simulink model "simulation"  (R2019b)
settings: Solver=ode45  StartTime=0.0  StopTime=10  FixedStep=0.001  RelTol=1e-9  AbsTol=1e-9
undefined symbols (not defined in the file or in its folder): K_int, modelData, MPC, pv0, ref
libraries: model_library x13, vrlib x7, sharedtransform x5, simulink x2
settings Model: PauseTimes=55  Creator=Matt  LastModifiedBy=Watson
settings SolverCC: MaxOrder=1  ZeroCrossAlgorithm=Adaptive
settings DataIOCC: SaveOutput=off  SignalLogging=off  DSMLogging=off  SaveTime=off  ReturnWorkspaceOutputs=off  StateSaveName=state
settings OptimizationCC: DefaultParameterBehavior=Inlined  UseDivisionForNetSlopeComputation=on  UseFloatMulNetSlope=on  InlineInvariantSignals=on  PassReuseOutputArgsAs=Individual arguments  ZeroExternalMemoryAtStartup=off  ZeroInternalMemoryAtStartup=off  NoFixptDivByZeroProtection=on  EfficientFloat2IntCast=on  LifeSpan=1  OptimizeBlockOrder=speed  DifferentSizesBufferReuse=on  EfficientTunableParamExpr=on
settings DebuggingCC: ReadBeforeWriteMsg=DisableAll  WriteAfterWriteMsg=DisableAll  WriteAfterReadMsg=DisableAll  MultiTaskDSMMsg=none  ParameterTunabilityLossMsg=error  RootOutportRequireBusObject=error  StrictBusMsg=ErrorOnBusTreatedAsVector  SFExecutionAtInitializationDiag=none  ArithmeticOperatorsInVariantConditions=warning
settings HardwareCC: ProdBitPerPointer=32  ProdBitPerSizeT=32  ProdBitPerPtrDiffT=32  ProdLargestAtomicInteger=Long  ProdWordSize=32  ProdLongLongMode=on  ProdHWDeviceType=ARM Compatible->ARM 9
settings ModelReferenceCC: UpdateModelReferenceTargets=IfOutOfDate
settings SFSimCC: SFSimEcho=off  SimUseLocalCustomCode=off  MATLABDynamicMemAlloc=off  CustomCodeUndefinedFunction=UseInterfaceOnly
settings RTWCC: SystemTargetFile=ert.tlc  TemplateMakefile=ert_default_tmf  GenerateReport=on  RTWUseLocalCustomCode=off  Toolchain=Microsoft Visual C++ 2015 v14.0 | nmake (64-bit Windows)  BuildConfiguration=Faster Runs  IncludeHyperlinkInReport=on  LaunchReport=on  GenerateTraceInfo=on  GenerateTraceReport=on  GenerateTraceReportSl=on  GenerateTraceReportSf=on  GenerateTraceReportEml=on  GenerateCodeMetricsReport=on
settings CodeAppCC: ForceParamTrailComments=on  IgnoreCustomStorageClasses=off  MaxIdLength=95  OperatorAnnotations=on  SimulinkDataObjDesc=on  SFDataObjDesc=on  CustomSymbolStrGlobalVar=rt$N$M  CustomSymbolStrType=$N$M  CustomSymbolStrFcn=$N$M$F  CustomSymbolStrMacro=$N$M  InsertBlockDesc=on
settings ERTTargetCC: GenerateSampleERTMain=on  IncludeMdlTerminateFcn=off  CombineSignalStateStructs=on  SupportComplex=off  SupportContinuousTime=on  SupportNonInlinedSFcns=on  InlinedParameterPlacement=NonHierarchical  ERTCustomFileTemplate=example_file_process.tlc  ERTFilePackagingFormat=CompactWithDataFile

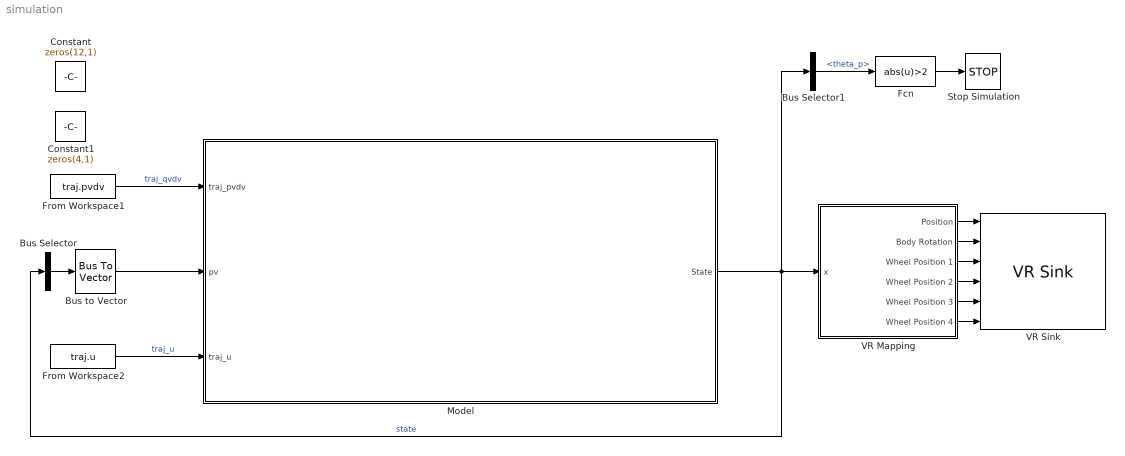
== system simulation ==
  Bus Selector : BusSelector  OutputSignals=x,y,phi,theta_p,vx,vy,dphi,dtheta_p  OutputAsBus=on
  Bus Selector1 : BusSelector  OutputSignals=theta_p
  Bus to Vector : BusToVector
  Constant : Constant  Value=zeros(12,1)
  Constant1 : Constant  Value=zeros(4,1)
  Fcn : Fcn  Expr=abs(u)>2
  From Workspace1 : FromWorkspace  VariableName=traj.pvdv  SampleTime=0  OutputAfterFinalValue=Holding final value
  From Workspace2 : FromWorkspace  VariableName=traj.u  SampleTime=0  OutputAfterFinalValue=Holding final value
  Model : Subsystem
  Stop Simulation : Stop
  VR Mapping : Subsystem
  VR Sink : vrlib/VR Sink  InstantiateOnLoad=on  SampleTime=0.01  ViewEnable=on  RemoteChange=off  RemoteView=off  FieldsWritten=Body_Position.translation.3.1.1.double#Body_Orientation.rotation.4.1.1.double#Wheel4.rotation.4.1.1.double#Wheel3.rotation.4.1.1.double#Wheel2.rotation.4.1.1.double#Wheel1.rotation.4.1.1.double  WorldFileName=3dworld.wrl  AutoView=off  VideoDimensions=[]  AllowVariableSize=off  FigureProperties="{'Position', 'Name', 'Viewpoint', 'CameraBound', 'CameraDirection', 'CameraPosition', 'CameraUpVector', 'ZoomFactor', 'Antialiasing', 'Headlight', 'Lighting', 'NavPanel', 'Sound', 'StatusBar', 'Stereo3D', 'Stereo3DCameraOffset', 'Stereo3DHIT', 'ToolBar', 'Textures', 'Transparency', 'Triad', 'Wireframe', 'NavZones', 'NavMode', 'NavSpeed', 'CaptureFileFormat', 'CaptureFileName', 'Record2DCompressMethod', 'Record2DCompressQuality', 'Record2D', 'Record2DFileName', 'Record2DFPS'; [1.0000000000000000e+00   7.6000000000000000e+01   1.9200000000000000e+03   9.1300000000000000e+02], '', '_untitled_2', 'on', [0.0000000000000000e+00   0.0000000000000000e+00  -1.0000000000000000e+00], [0.0000000000000000e+00   0.0000000000000000e+00   0.0000000000000000e+00], [0.0000000000000000e+00   1.0000000000000000e+00   0.0000000000000000e+00], [1.0000000000000000e+00], 'on', 'on', 'on', 'halfbar', 'on', 'on', 'off', [1.0000000149011612e-01], [0.0000000000000000e+00], 'on', 'on', 'on', 'none', 'off', 'off', 'fly', 'normal', 'tif', '%f_anim_%n.tif', 'auto', [7.5000000000000000e+01], 'off', '%f_anim_%n.avi', 'auto'}"
      settings: SourceProductBaseCode=VR
  wires:
  Model/1(State) -> Bus Selector1/1, VR Mapping/1(x), Bus Selector/1  "state"
  Bus Selector/1 -> Bus to Vector/1
  VR Mapping/1(Position) -> VR Sink/1
  VR Mapping/2(Body Rotation) -> VR Sink/2
  VR Mapping/3(Wheel Position 1) -> VR Sink/3
  VR Mapping/4(Wheel Position 2) -> VR Sink/4
  VR Mapping/5(Wheel Position 3) -> VR Sink/5
  VR Mapping/6(Wheel Position 4) -> VR Sink/6
  Bus to Vector/1 -> Model/2(pv)
  From Workspace1/1 -> Model/1(traj_pvdv)  "traj_qvdv"
  From Workspace2/1 -> Model/3(traj_u)  "traj_u"
  Bus Selector1/1 -> Fcn/1  "<theta_p>"
  Fcn/1 -> Stop Simulation/1

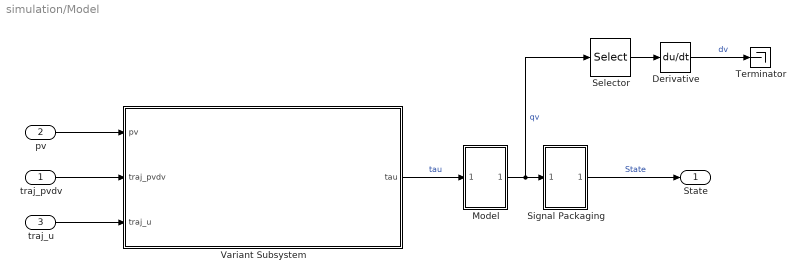
== system simulation/Model ==
  traj_pvdv : Inport
  pv : Inport  Port=2
  traj_u : Inport  Port=3
  Derivative : Derivative
  Model : Subsystem
  Selector : Selector  InputPortWidth=8  IndexOptions=Index vector (dialog)  Indices=[5:8]  OutputSizes=1
  Signal Packaging : Subsystem
  Terminator : Terminator
  Variant Subsystem : Subsystem  VariantControlMode=Label  Variant=on  LabelModeActiveChoice=LQR
  State : Outport  VectorParamsAs1DForOutWhenUnconnected=off
  wires:
  Model/1("[q;v]") -> Selector/1, Signal Packaging/1(In1)  "qv"
  Signal Packaging/1(Out1) -> State/1  "State"
  traj_pvdv/1 -> Variant Subsystem/2(traj_pvdv)
  traj_u/1 -> Variant Subsystem/3(traj_u)
  Selector/1 -> Derivative/1
  Derivative/1 -> Terminator/1  "dv"
  pv/1 -> Variant Subsystem/1(pv)
  Variant Subsystem/1(tau) -> Model/1(tau)  "tau"

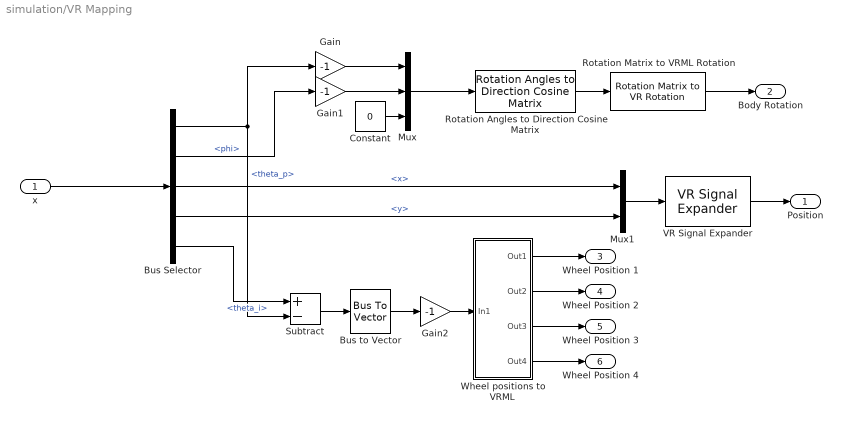
== system simulation/VR Mapping ==
  x : Inport
  Bus Selector : BusSelector  OutputSignals=theta_p,phi,x,y,theta_i
  Bus to Vector : BusToVector
  Constant : Constant  Value=0
  Gain : Gain  Gain=-1
  Gain1 : Gain  Gain=-1
  Gain2 : Gain  Gain=-1
  Mux : Mux  Inputs=3
  Mux1 : Mux  Inputs=2
  Rotation Angles to Direction Cosine Matrix : sharedtransform/Rotation Angles to Direction Cosine Matrix  rotationOrder=XZY  aMode=aMode
      settings: SourceProductBaseCode=AE
  Rotation Matrix to VRML Rotation : vrlib/Utilities/Rotation Matrix to VR Rotation  maxzero=1e-12
      settings: SourceProductName=Simulink 3D Animation  SourceProductBaseCode=VR
  Subtract : Sum  Inputs=+-
  VR Signal Expander : vrlib/VR Signal Expander  outwidth=3  outidx=[1 2]
      settings: SourceProductName=Simulink 3D Animation  SourceProductBaseCode=VR
  Wheel positions to VRML : Subsystem
  Position : Outport  VectorParamsAs1DForOutWhenUnconnected=off
  Body Rotation : Outport  Port=2  VectorParamsAs1DForOutWhenUnconnected=off
  Wheel Position 1 : Outport  Port=3  VectorParamsAs1DForOutWhenUnconnected=off
  Wheel Position 2 : Outport  Port=4  VectorParamsAs1DForOutWhenUnconnected=off
  Wheel Position 3 : Outport  Port=5  VectorParamsAs1DForOutWhenUnconnected=off
  Wheel Position 4 : Outport  Port=6  VectorParamsAs1DForOutWhenUnconnected=off
  wires:
  Mux/1 -> Rotation Angles to Direction Cosine Matrix/1
  Rotation Angles to Direction Cosine Matrix/1 -> Rotation Matrix to VRML Rotation/1
  Rotation Matrix to VRML Rotation/1 -> Body Rotation/1
  Constant/1 -> Mux/3
  VR Signal Expander/1 -> Position/1
  Mux1/1 -> VR Signal Expander/1
  Bus Selector/1 -> Subtract/2, Gain/1  "<theta_p>"
  Bus Selector/2 -> Gain1/1  "<phi>"
  Bus Selector/3 -> Mux1/1  "<x>"
  Bus Selector/4 -> Mux1/2  "<y>"
  Bus to Vector/1 -> Gain2/1
  Subtract/1 -> Bus to Vector/1
  Bus Selector/5 -> Subtract/1  "<theta_i>"
  Gain/1 -> Mux/1
  Gain1/1 -> Mux/2
  Gain2/1 -> Wheel positions to VRML/1(In1)
  x/1 -> Bus Selector/1
  Wheel positions to VRML/1(Out1) -> Wheel Position 1/1
  Wheel positions to VRML/2(Out2) -> Wheel Position 2/1
  Wheel positions to VRML/3(Out3) -> Wheel Position 3/1
  Wheel positions to VRML/4(Out4) -> Wheel Position 4/1

== system simulation/Model/Model ==
  tau : Inport
  Integrator2 : Integrator  InitialCondition=pv0
  dynamics_dqdv : model_library/dynamics_dqdv  SystemSampleTime=-1  Latency=0  AutoFrameSizeCalculation=off
  "[q;v]" : Outport  VectorParamsAs1DForOutWhenUnconnected=off
  wires:
  Integrator2/1 -> dynamics_dqdv/1, "[q;v]"/1
  dynamics_dqdv/1 -> Integrator2/1  "dqdv"
  tau/1 -> dynamics_dqdv/2

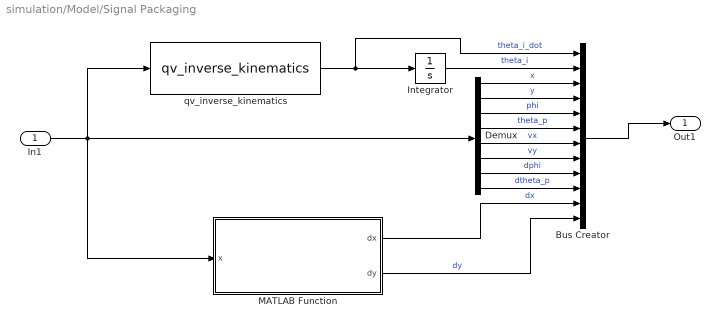
== system simulation/Model/Signal Packaging ==
  In1 : Inport
  Bus Creator : BusCreator  Inputs=12
  Demux : Demux  Outputs=8
  Integrator : Integrator  InitialCondition=[0 0 0 0]
  MATLAB Function : MATLAB Function  TreatAsAtomicUnit=on
  qv_inverse_kinematics : model_library/qv_inverse_kinematics  SystemSampleTime=-1  Latency=0  AutoFrameSizeCalculation=off
  Out1 : Outport  VectorParamsAs1DForOutWhenUnconnected=off
  wires:
  Demux/1 -> Bus Creator/3  "x"
  Demux/6 -> Bus Creator/8  "vy"
  Demux/3 -> Bus Creator/5  "phi"
  Demux/7 -> Bus Creator/9  "dphi"
  qv_inverse_kinematics/1 -> Integrator/1, Bus Creator/1  "theta_i_dot"
  Demux/8 -> Bus Creator/10  "dtheta_p"
  In1/1 -> MATLAB Function/1(x), Demux/1, qv_inverse_kinematics/1
  Demux/2 -> Bus Creator/4  "y"
  Demux/4 -> Bus Creator/6  "theta_p"
  Demux/5 -> Bus Creator/7  "vx"
  Integrator/1 -> Bus Creator/2  "theta_i"
  Bus Creator/1 -> Out1/1
  MATLAB Function/1(dx) -> Bus Creator/11  "dx"
  MATLAB Function/2(dy) -> Bus Creator/12  "dy"

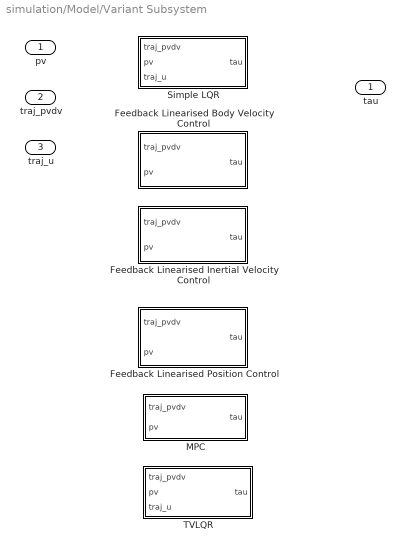
== system simulation/Model/Variant Subsystem ==
  pv : Inport
  traj_pvdv : Inport  Port=2
  traj_u : Inport  Port=3
  Feedback Linearised Body Velocity Control : Subsystem  VariantControl=FeedbackLinearisedBodyVelocity
  Feedback Linearised Inertial Velocity Control : Subsystem  VariantControl=FeedbackLinearisedInertialVelocity
  Feedback Linearised Position Control : Subsystem  VariantControl=FeedbackLinearisedPosition
  MPC : Subsystem  VariantControl=Variant
  Simple LQR : Subsystem  VariantControl=LQR
  TVLQR : Subsystem  VariantControl=TVLQR
  tau : Outport  VectorParamsAs1DForOutWhenUnconnected=off

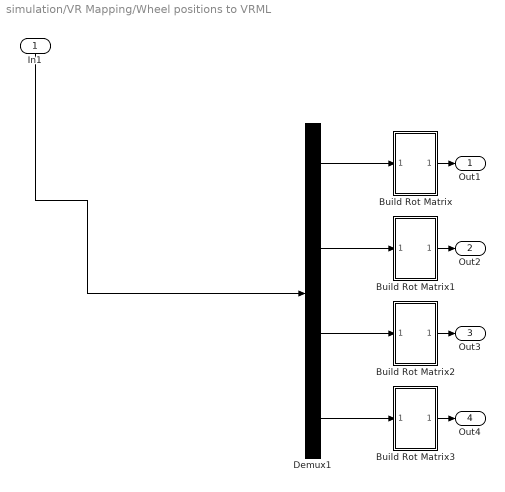
== system simulation/VR Mapping/Wheel positions to VRML ==
  In1 : Inport
  Build Rot Matrix : Subsystem
  Build Rot Matrix1 : Subsystem
  Build Rot Matrix2 : Subsystem
  Build Rot Matrix3 : Subsystem
  Demux1 : Demux
  Out1 : Outport  VectorParamsAs1DForOutWhenUnconnected=off
  Out2 : Outport  Port=2  VectorParamsAs1DForOutWhenUnconnected=off
  Out3 : Outport  Port=3  VectorParamsAs1DForOutWhenUnconnected=off
  Out4 : Outport  Port=4  VectorParamsAs1DForOutWhenUnconnected=off
  wires:
  Demux1/3 -> Build Rot Matrix2/1(In1)
  Build Rot Matrix1/1(Out1) -> Out2/1
  Build Rot Matrix3/1(Out1) -> Out4/1
  Build Rot Matrix2/1(Out1) -> Out3/1
  In1/1 -> Demux1/1
  Demux1/2 -> Build Rot Matrix1/1(In1)
  Demux1/4 -> Build Rot Matrix3/1(In1)
  Demux1/1 -> Build Rot Matrix/1(In1)
  Build Rot Matrix/1(Out1) -> Out1/1

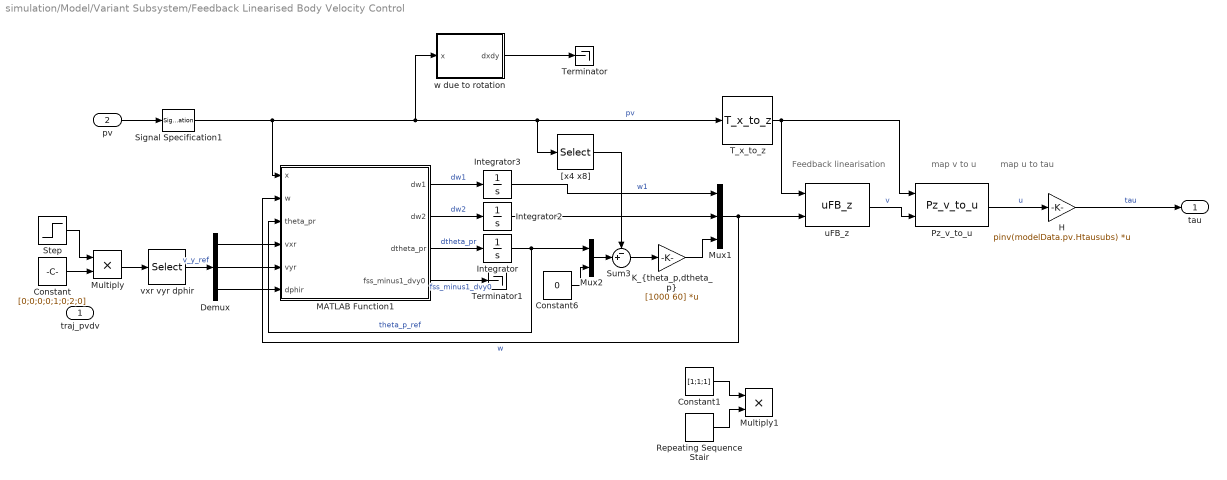
== system simulation/Model/Variant Subsystem/Feedback Linearised Body Velocity Control ==
  note: Feedback linearisation
  note: map v to u
  note: map u to tau
  traj_pvdv : Inport
  pv : Inport  Port=2
  Constant : Constant  Value=[0;0;0;0;1;0;2;0]
  Constant1 : Constant  Value=[1;1;1]
  Constant6 : Constant  Value=0
  Demux : Demux  Outputs=3
  H : Gain  Gain=pinv(modelData.pv.Htausubs)  Multiplication=Matrix(K*u)
  Integrator : Integrator  InitialCondition=pv0(4)
  Integrator2 : Integrator
  Integrator3 : Integrator
  "K_{theta_p,dtheta_p}" : Gain  Gain=[1000 60]  Multiplication=Matrix(K*u)
  MATLAB Function1 : MATLAB Function  TreatAsAtomicUnit=on
  Multiply : Product
  Multiply1 : Product
  Mux1 : Mux  Inputs=3
  Mux2 : Mux  Inputs=2
  Pz_v_to_u : model_library/Pz_v_to_u  SystemSampleTime=-1  Latency=0  AutoFrameSizeCalculation=off
  Repeating Sequence Stair : simulink/Sources/Repeating Sequence Stair  OutValues=[1 -1 -1 1]  tsamp=1  OutMin=[]  OutMax=[]  OutDataTypeStr=double  OutputDataTypeScalingMode=double  OutDataType=fixdt(0,8)  ConRadixGroup=Best Precision: Vector-wise  OutScaling=2^-12
  Signal Specification1 : SignalSpecification  Dimensions=[8 1]
  Step : Step  SampleTime=0
  Sum3 : Sum  Inputs=-+|
  T_x_to_z : model_library/T_x_to_z  SystemSampleTime=-1  Latency=0  AutoFrameSizeCalculation=off
  Terminator : Terminator
  Terminator1 : Terminator
  "[x4 x8]" : Selector  InputPortWidth=8  IndexOptions=Index vector (dialog)  Indices=[4 8]  OutputSizes=1
  uFB_z : model_library/uFB_z  SystemSampleTime=-1  Latency=0  AutoFrameSizeCalculation=off
  vxr vyr dphir : Selector  InputPortWidth=8  IndexOptions=Index vector (dialog)  Indices=5:7  OutputSizes=1
  w due to rotation : MATLAB Function  TreatAsAtomicUnit=on
  tau : Outport  VectorParamsAs1DForOutWhenUnconnected=off
  wires:
  T_x_to_z/1 -> uFB_z/1, Pz_v_to_u/1
  Sum3/1 -> "K_{theta_p,dtheta_p}"/1
  uFB_z/1 -> Pz_v_to_u/2  "v"
  "[x4 x8]"/1 -> Sum3/1
  pv/1 -> Signal Specification1/1
  Signal Specification1/1 -> MATLAB Function1/1(x), w due to rotation/1(x), T_x_to_z/1, "[x4 x8]"/1  "pv"
  H/1 -> tau/1  "tau"
  Mux2/1 -> Sum3/2
  Demux/2 -> MATLAB Function1/5(vyr)
  Demux/1 -> MATLAB Function1/4(vxr)
  Demux/3 -> MATLAB Function1/6(dphir)
  vxr vyr dphir/1 -> Demux/1  "v_y_ref"
  MATLAB Function1/3(dtheta_pr) -> Integrator/1  "dtheta_pr"
  MATLAB Function1/1(dw1) -> Integrator3/1  "dw1"
  MATLAB Function1/2(dw2) -> Integrator2/1  "dw2"
  "K_{theta_p,dtheta_p}"/1 -> Mux1/3
  Pz_v_to_u/1 -> H/1  "u"
  Integrator2/1 -> Mux1/2
  Mux1/1 -> uFB_z/2, MATLAB Function1/2(w)  "w"
  Constant6/1 -> Mux2/2
  Integrator3/1 -> Mux1/1  "w1"
  Integrator/1 -> MATLAB Function1/3(theta_pr), Mux2/1  "theta_p_ref"
  w due to rotation/1(dxdy) -> Terminator/1
  MATLAB Function1/4(fss_minus1_dvy0) -> Terminator1/1  "fss_minus1_dvy0"
  Constant/1 -> Multiply/2
  Multiply/1 -> vxr vyr dphir/1
  Step/1 -> Multiply/1
  Repeating Sequence Stair/1 -> Multiply1/2
  Constant1/1 -> Multiply1/1

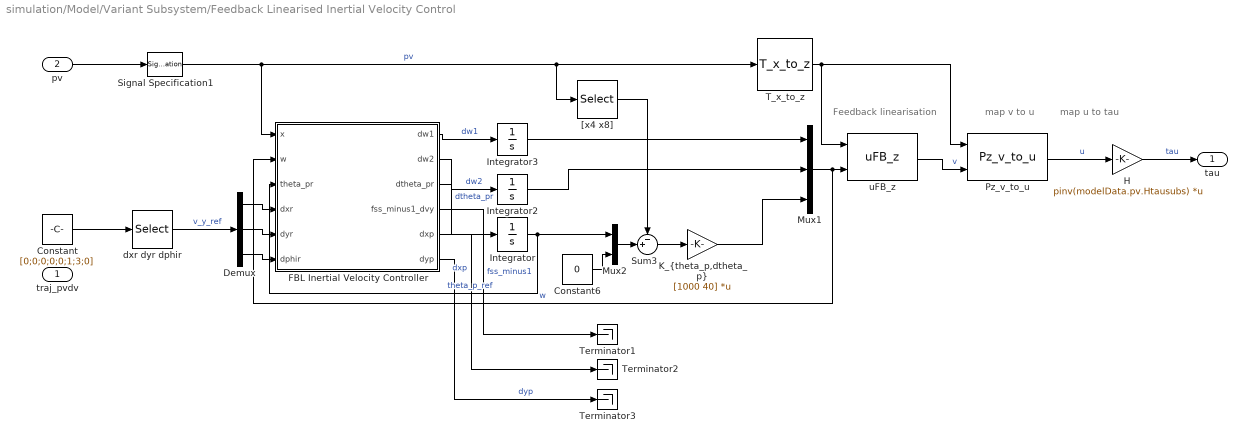
== system simulation/Model/Variant Subsystem/Feedback Linearised Inertial Velocity Control ==
  note: Feedback linearisation
  note: map v to u
  note: map u to tau
  traj_pvdv : Inport
  pv : Inport  Port=2
  Constant : Constant  Value=[0;0;0;0;0;1;3;0]
  Constant6 : Constant  Value=0
  Demux : Demux  Outputs=3
  FBL Inertial Velocity Controller : MATLAB Function  TreatAsAtomicUnit=on
  H : Gain  Gain=pinv(modelData.pv.Htausubs)  Multiplication=Matrix(K*u)
  Integrator : Integrator
  Integrator2 : Integrator
  Integrator3 : Integrator
  "K_{theta_p,dtheta_p}" : Gain  Gain=[1000 40]  Multiplication=Matrix(K*u)
  Mux1 : Mux  Inputs=3
  Mux2 : Mux  Inputs=2
  Pz_v_to_u : model_library/Pz_v_to_u  SystemSampleTime=-1  Latency=0  AutoFrameSizeCalculation=off
  Signal Specification1 : SignalSpecification  Dimensions=[8 1]
  Sum3 : Sum  Inputs=-+|
  T_x_to_z : model_library/T_x_to_z  SystemSampleTime=-1  Latency=0  AutoFrameSizeCalculation=off
  Terminator1 : Terminator
  Terminator2 : Terminator
  Terminator3 : Terminator
  "[x4 x8]" : Selector  InputPortWidth=8  IndexOptions=Index vector (dialog)  Indices=[4 8]  OutputSizes=1
  dxr dyr dphir : Selector  InputPortWidth=8  IndexOptions=Index vector (dialog)  Indices=5:7  OutputSizes=1
  uFB_z : model_library/uFB_z  SystemSampleTime=-1  Latency=0  AutoFrameSizeCalculation=off
  tau : Outport  VectorParamsAs1DForOutWhenUnconnected=off
  wires:
  T_x_to_z/1 -> uFB_z/1, Pz_v_to_u/1
  Sum3/1 -> "K_{theta_p,dtheta_p}"/1
  "[x4 x8]"/1 -> Sum3/1
  pv/1 -> Signal Specification1/1
  Signal Specification1/1 -> T_x_to_z/1, "[x4 x8]"/1, FBL Inertial Velocity Controller/1(x)  "pv"
  H/1 -> tau/1  "tau"
  Mux2/1 -> Sum3/2
  Constant/1 -> dxr dyr dphir/1
  Demux/2 -> FBL Inertial Velocity Controller/5(dyr)
  Demux/1 -> FBL Inertial Velocity Controller/4(dxr)
  Demux/3 -> FBL Inertial Velocity Controller/6(dphir)
  dxr dyr dphir/1 -> Demux/1  "v_y_ref"
  FBL Inertial Velocity Controller/2(dw2) -> Integrator2/1  "dw2"
  FBL Inertial Velocity Controller/1(dw1) -> Integrator3/1  "dw1"
  Mux1/1 -> FBL Inertial Velocity Controller/2(w), uFB_z/2  "w"
  uFB_z/1 -> Pz_v_to_u/2  "v"
  Pz_v_to_u/1 -> H/1  "u"
  Integrator2/1 -> Mux1/2
  Integrator3/1 -> Mux1/1
  FBL Inertial Velocity Controller/3(dtheta_pr) -> Integrator/1  "dtheta_pr"
  "K_{theta_p,dtheta_p}"/1 -> Mux1/3
  Integrator/1 -> FBL Inertial Velocity Controller/3(theta_pr), Mux2/1  "theta_p_ref"
  Constant6/1 -> Mux2/2
  FBL Inertial Velocity Controller/4(fss_minus1_dvy) -> Terminator1/1  "fss_minus1"
  FBL Inertial Velocity Controller/5(dxp) -> Terminator2/1  "dxp"
  FBL Inertial Velocity Controller/6(dyp) -> Terminator3/1  "dyp"

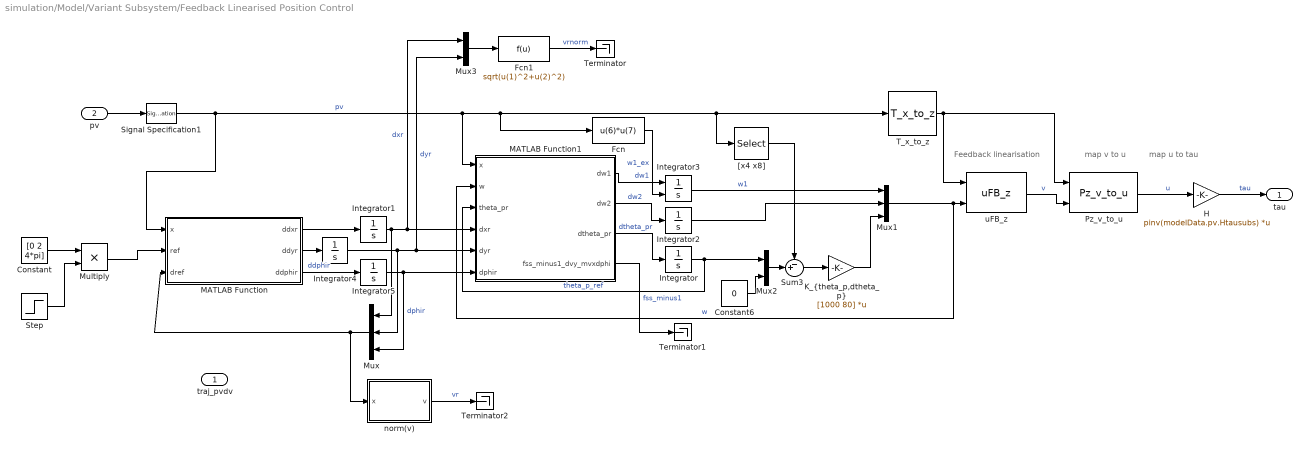
== system simulation/Model/Variant Subsystem/Feedback Linearised Position Control ==
  note: Feedback linearisation
  note: map v to u
  note: map u to tau
  traj_pvdv : Inport
  pv : Inport  Port=2
  Constant : Constant  Value=[0 2 4*pi]
  Constant6 : Constant  Value=0
  Fcn : Fcn  Expr=u(6)*u(7)
  Fcn1 : Fcn  Expr=sqrt(u(1)^2+u(2)^2)
  H : Gain  Gain=pinv(modelData.pv.Htausubs)  Multiplication=Matrix(K*u)
  Integrator : Integrator  InitialCondition=pv0(4)
  Integrator{1..2,4..5} (4 alike) : Integrator
  Integrator3 : Integrator  InitialConditionSource=external
  "K_{theta_p,dtheta_p}" : Gain  Gain=[1000 80]  Multiplication=Matrix(K*u)
  MATLAB Function : MATLAB Function  TreatAsAtomicUnit=on
  MATLAB Function1 : MATLAB Function  TreatAsAtomicUnit=on
  Multiply : Product
  Mux : Mux  Inputs=3
  Mux1 : Mux  Inputs=3
  Mux2 : Mux  Inputs=2
  Mux3 : Mux  Inputs=2
  Pz_v_to_u : model_library/Pz_v_to_u  SystemSampleTime=-1  Latency=0  AutoFrameSizeCalculation=off
  Signal Specification1 : SignalSpecification  Dimensions=[8 1]
  Step : Step  Time=2  SampleTime=0
  Sum3 : Sum  Inputs=-+|
  T_x_to_z : model_library/T_x_to_z  SystemSampleTime=-1  Latency=0  AutoFrameSizeCalculation=off
  Terminator : Terminator
  Terminator1 : Terminator
  Terminator2 : Terminator
  "[x4 x8]" : Selector  InputPortWidth=8  IndexOptions=Index vector (dialog)  Indices=[4 8]  OutputSizes=1
  norm(v) : MATLAB Function  TreatAsAtomicUnit=on
  uFB_z : model_library/uFB_z  SystemSampleTime=-1  Latency=0  AutoFrameSizeCalculation=off
  tau : Outport  VectorParamsAs1DForOutWhenUnconnected=off
  wires:
  MATLAB Function/1(ddxr) -> Integrator1/1
  MATLAB Function/3(ddphir) -> Integrator5/1  "ddphir"
  Integrator2/1 -> Mux1/2
  "[x4 x8]"/1 -> Sum3/1
  uFB_z/1 -> Pz_v_to_u/2  "v"
  Sum3/1 -> "K_{theta_p,dtheta_p}"/1
  T_x_to_z/1 -> uFB_z/1, Pz_v_to_u/1
  Signal Specification1/1 -> MATLAB Function/1(x), T_x_to_z/1, "[x4 x8]"/1, Fcn/1, MATLAB Function1/1(x)  "pv"
  MATLAB Function1/2(dw2) -> Integrator2/1  "dw2"
  "K_{theta_p,dtheta_p}"/1 -> Mux1/3
  H/1 -> tau/1  "tau"
  Fcn/1 -> Integrator3/2  "w1_ex"
  Integrator3/1 -> Mux1/1  "w1"
  pv/1 -> Signal Specification1/1
  Pz_v_to_u/1 -> H/1  "u"
  Integrator/1 -> MATLAB Function1/3(theta_pr), Mux2/1  "theta_p_ref"
  Mux2/1 -> Sum3/2
  MATLAB Function1/1(dw1) -> Integrator3/1  "dw1"
  Constant6/1 -> Mux2/2
  Mux1/1 -> MATLAB Function1/2(w), uFB_z/2  "w"
  MATLAB Function1/3(dtheta_pr) -> Integrator/1  "dtheta_pr"
  MATLAB Function/2(ddyr) -> Integrator4/1
  Integrator1/1 -> Mux/1, Mux3/1, MATLAB Function1/4(dxr)  "dxr"
  Integrator4/1 -> Mux/2, Mux3/2, MATLAB Function1/5(dyr)  "dyr"
  Integrator5/1 -> Mux/3, MATLAB Function1/6(dphir)  "dphir"
  Fcn1/1 -> Terminator/1  "vrnorm"
  Mux3/1 -> Fcn1/1
  MATLAB Function1/4(fss_minus1_dvy_mvxdphi) -> Terminator1/1  "fss_minus1"
  Mux/1 -> norm(v)/1(x), MATLAB Function/3(dref)
  norm(v)/1(v) -> Terminator2/1  "vr"
  Constant/1 -> Multiply/1
  Step/1 -> Multiply/2
  Multiply/1 -> MATLAB Function/2(ref)

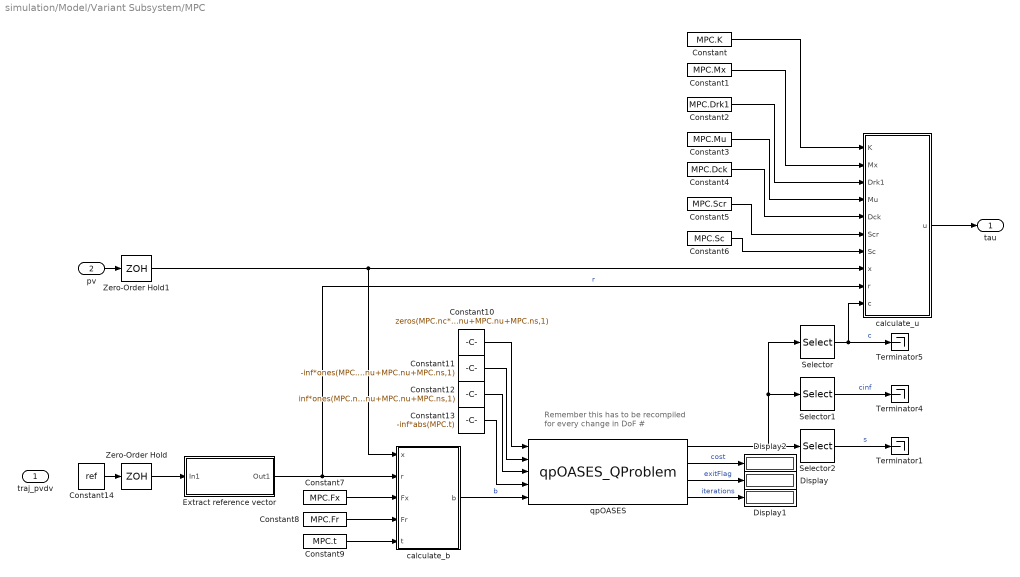
== system simulation/Model/Variant Subsystem/MPC ==
  note: Remember this has to be recompiled
      | for every change in DoF #
  traj_pvdv : Inport
  pv : Inport  Port=2
  Constant : Constant  Value=MPC.K
  Constant1 : Constant  Value=MPC.Mx
  Constant10 : Constant  Value=zeros(MPC.nc*MPC.nu+MPC.nu+MPC.ns,1)
  Constant11 : Constant  Value=-inf*ones(MPC.nc*MPC.nu+MPC.nu+MPC.ns,1)
  Constant12 : Constant  Value=inf*ones(MPC.nc*MPC.nu+MPC.nu+MPC.ns,1)
  Constant13 : Constant  Value=-inf*abs(MPC.t)
  Constant14 : Constant  Value=ref
  Constant2 : Constant  Value=MPC.Drk1
  Constant3 : Constant  Value=MPC.Mu
  Constant4 : Constant  Value=MPC.Dck
  Constant5 : Constant  Value=MPC.Scr
  Constant6 : Constant  Value=MPC.Sc
  Constant7 : Constant  Value=MPC.Fx
  Constant8 : Constant  Value=MPC.Fr
  Constant9 : Constant  Value=MPC.t
  Display : Display
  Display1 : Display
  Display2 : Display
  Extract reference vector : Subsystem
  Selector : Selector  InputPortWidth=MPC.nc*MPC.nu + MPC.nu + MPC.ns  IndexOptions=Index vector (dialog)  Indices=[1:MPC.nc*MPC.nu]  OutputSizes=1
  Selector1 : Selector  InputPortWidth=MPC.nc*MPC.nu + MPC.nu + MPC.ns  IndexOptions=Index vector (dialog)  Indices=[1+MPC.nc*MPC.nu:MPC.nc*MPC.nu+MPC.nu]  OutputSizes=1
  Selector2 : Selector  InputPortWidth=MPC.nc*MPC.nu + MPC.nu + MPC.ns  IndexOptions=Index vector (dialog)  Indices=[1+MPC.nc*MPC.nu+MPC.nu:MPC.nc*MPC.nu+MPC.nu+MPC.ns]  OutputSizes=1
  Terminator1 : Terminator
  Terminator4 : Terminator
  Terminator5 : Terminator
  Zero-Order Hold : ZeroOrderHold  SampleTime=MPC.Ts
  Zero-Order Hold1 : ZeroOrderHold  SampleTime=MPC.Ts
  calculate_b : MATLAB Function  TreatAsAtomicUnit=on
  calculate_u : MATLAB Function  TreatAsAtomicUnit=on
  qpOASES : S-Function  FunctionName=qpOASES_QProblem  Parameters=MPC.H,MPC.A  SFunctionDeploymentMode=off  EnableBusSupport=off
  tau : Outport  VectorParamsAs1DForOutWhenUnconnected=off
  wires:
  Constant13/1 -> qpOASES/4
  Constant2/1 -> calculate_u/3(Drk1)
  Constant3/1 -> calculate_u/4(Mu)
  Constant11/1 -> qpOASES/2
  Extract reference vector/1(Out1) -> calculate_u/9(r), calculate_b/2(r)  "r"
  qpOASES/2 -> Display2/1  "cost"
  Constant4/1 -> calculate_u/5(Dck)
  Selector1/1 -> Terminator4/1  "cinf"
  calculate_u/1(u) -> tau/1
  Constant10/1 -> qpOASES/1
  calculate_b/1(b) -> qpOASES/5  "b"
  Constant7/1 -> calculate_b/3(Fx)
  Constant1/1 -> calculate_u/2(Mx)
  Constant8/1 -> calculate_b/4(Fr)
  qpOASES/3 -> Display/1  "exitFlag"
  Constant/1 -> calculate_u/1(K)
  Constant6/1 -> calculate_u/7(Sc)
  qpOASES/4 -> Display1/1  "iterations"
  qpOASES/1 -> Selector2/1, Selector1/1, Selector/1
  Constant5/1 -> calculate_u/6(Scr)
  Selector/1 -> Terminator5/1, calculate_u/10(c)  "c"
  Selector2/1 -> Terminator1/1  "s"
  pv/1 -> Zero-Order Hold1/1
  Constant12/1 -> qpOASES/3
  Constant9/1 -> calculate_b/5(t)
  Constant14/1 -> Zero-Order Hold/1
  Zero-Order Hold/1 -> Extract reference vector/1(In1)
  Zero-Order Hold1/1 -> calculate_b/1(x), calculate_u/8(x)

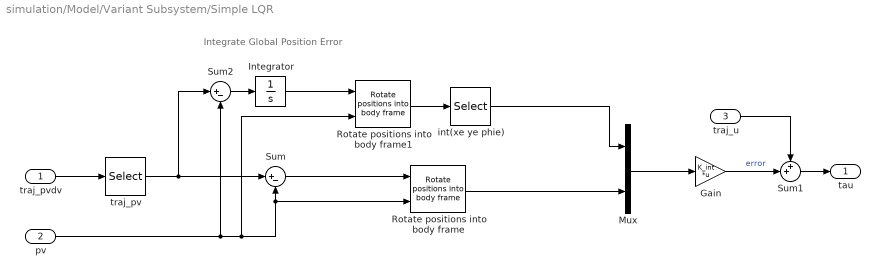
== system simulation/Model/Variant Subsystem/Simple LQR ==
  note: Integrate Global Position Error
  traj_pvdv : Inport
  pv : Inport  Port=2
  traj_u : Inport  Port=3
  Gain : Gain  Gain=K_int  Multiplication=Matrix(K*u)
  Integrator : Integrator  InitialCondition=zeros(8,1)
  Mux : Mux  Inputs=2
  Rotate positions into body frame : model_library/Rotate positions into body frame  SystemSampleTime=-1  Latency=0  AutoFrameSizeCalculation=off
  Rotate positions into body frame1 : model_library/Rotate positions into body frame  SystemSampleTime=-1  Latency=0  AutoFrameSizeCalculation=off
  Sum : Sum  Inputs=|+-
  Sum1 : Sum  Inputs=++|
  Sum2 : Sum  Inputs=|+-
  int(xe ye phie) : Selector  InputPortWidth=8  IndexOptions=Index vector (dialog)  Indices=[1:3]  OutputSizes=1
  traj_pv : Selector  InputPortWidth=12  IndexOptions=Index vector (dialog)  Indices=[1:8]  OutputSizes=1
  tau : Outport  VectorParamsAs1DForOutWhenUnconnected=off
  wires:
  Gain/1 -> Sum1/2  "error"
  traj_u/1 -> Sum1/1
  Sum1/1 -> tau/1
  Sum/1 -> Rotate positions into body frame/1
  Sum2/1 -> Integrator/1
  Rotate positions into body frame1/1 -> int(xe ye phie)/1
  Integrator/1 -> Rotate positions into body frame1/1
  Rotate positions into body frame/1 -> Mux/2
  int(xe ye phie)/1 -> Mux/1
  traj_pvdv/1 -> traj_pv/1
  pv/1 -> Rotate positions into body frame1/2, Rotate positions into body frame/2, Sum/2, Sum2/2
  Mux/1 -> Gain/1
  traj_pv/1 -> Sum2/1, Sum/1

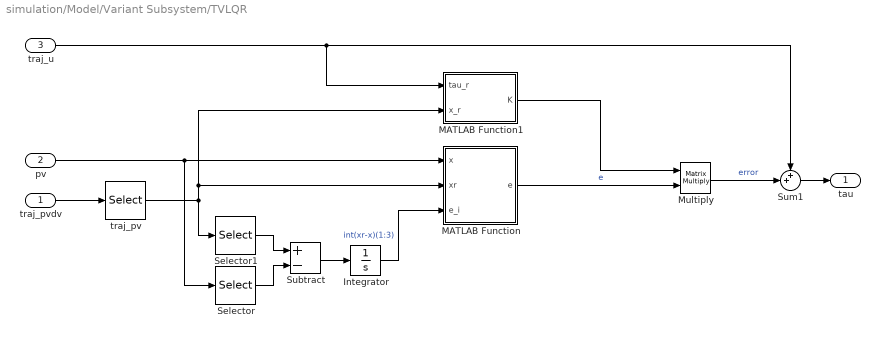
== system simulation/Model/Variant Subsystem/TVLQR ==
  traj_pvdv : Inport
  pv : Inport  Port=2
  traj_u : Inport  Port=3
  Integrator : Integrator  InitialCondition=zeros(3,1)
  MATLAB Function : MATLAB Function  TreatAsAtomicUnit=on
  MATLAB Function1 : MATLAB Function  TreatAsAtomicUnit=on  SystemSampleTime=0.01
  Multiply : Product  Multiplication=Matrix(*)
  Selector : Selector  InputPortWidth=8  IndexOptions=Index vector (dialog)  Indices=[1:3]  OutputSizes=1
  Selector1 : Selector  InputPortWidth=8  IndexOptions=Index vector (dialog)  Indices=[1:3]  OutputSizes=1
  Subtract : Sum  Inputs=+-
  Sum1 : Sum  Inputs=++|
  traj_pv : Selector  InputPortWidth=12  IndexOptions=Index vector (dialog)  Indices=[1:8]  OutputSizes=1
  tau : Outport  VectorParamsAs1DForOutWhenUnconnected=off
  wires:
  Multiply/1 -> Sum1/2  "error"
  Sum1/1 -> tau/1
  traj_pvdv/1 -> traj_pv/1
  pv/1 -> MATLAB Function/1(x), Selector/1
  traj_pv/1 -> Selector1/1, MATLAB Function1/2(x_r), MATLAB Function/2(xr)
  traj_u/1 -> MATLAB Function1/1(tau_r), Sum1/1
  MATLAB Function1/1(K) -> Multiply/1
  MATLAB Function/1(e) -> Multiply/2  "e"
  Selector1/1 -> Subtract/1
  Selector/1 -> Subtract/2
  Subtract/1 -> Integrator/1
  Integrator/1 -> MATLAB Function/3(e_i)  "int(xr-x)(1:3)"

== system simulation/VR Mapping/Wheel positions to VRML/Build Rot Matrix ==
  In1 : Inport
  Constant1 : Constant  Value=pi/2
  Constant2 : Constant  Value=pi/2
  Mux : Mux  Inputs=3
  Rotation Angles to Direction Cosine Matrix : sharedtransform/Rotation Angles to Direction Cosine Matrix  rotationOrder=YZX  aMode=aMode
      settings: SourceProductBaseCode=AE
  Rotation Matrix to VRML Rotation1 : vrlib/Utilities/Rotation Matrix to VR Rotation  maxzero=1e-12
      settings: SourceProductName=Simulink 3D Animation  SourceProductBaseCode=VR
  Out1 : Outport  VectorParamsAs1DForOutWhenUnconnected=off
  wires:
  In1/1 -> Mux/1
  Mux/1 -> Rotation Angles to Direction Cosine Matrix/1
  Constant1/1 -> Mux/2
  Constant2/1 -> Mux/3
  Rotation Angles to Direction Cosine Matrix/1 -> Rotation Matrix to VRML Rotation1/1
  Rotation Matrix to VRML Rotation1/1 -> Out1/1

== system simulation/VR Mapping/Wheel positions to VRML/Build Rot Matrix1 ==
  In1 : Inport
  Constant1 : Constant  Value=pi/2
  Constant2 : Constant  Value=pi/2
  Mux : Mux  Inputs=3
  Rotation Angles to Direction Cosine Matrix : sharedtransform/Rotation Angles to Direction Cosine Matrix  rotationOrder=YZX  aMode=aMode
      settings: SourceProductBaseCode=AE
  Rotation Matrix to VRML Rotation1 : vrlib/Utilities/Rotation Matrix to VR Rotation  maxzero=1e-12
      settings: SourceProductName=Simulink 3D Animation  SourceProductBaseCode=VR
  Out1 : Outport  VectorParamsAs1DForOutWhenUnconnected=off
  wires:
  In1/1 -> Mux/1
  Mux/1 -> Rotation Angles to Direction Cosine Matrix/1
  Constant1/1 -> Mux/2
  Constant2/1 -> Mux/3
  Rotation Angles to Direction Cosine Matrix/1 -> Rotation Matrix to VRML Rotation1/1
  Rotation Matrix to VRML Rotation1/1 -> Out1/1

== system simulation/VR Mapping/Wheel positions to VRML/Build Rot Matrix2 ==
  In1 : Inport
  Constant1 : Constant  Value=pi/2
  Constant2 : Constant  Value=pi/2
  Mux : Mux  Inputs=3
  Rotation Angles to Direction Cosine Matrix : sharedtransform/Rotation Angles to Direction Cosine Matrix  rotationOrder=YZX  aMode=aMode
      settings: SourceProductBaseCode=AE
  Rotation Matrix to VRML Rotation1 : vrlib/Utilities/Rotation Matrix to VR Rotation  maxzero=1e-12
      settings: SourceProductName=Simulink 3D Animation  SourceProductBaseCode=VR
  Out1 : Outport  VectorParamsAs1DForOutWhenUnconnected=off
  wires:
  In1/1 -> Mux/1
  Mux/1 -> Rotation Angles to Direction Cosine Matrix/1
  Constant1/1 -> Mux/2
  Constant2/1 -> Mux/3
  Rotation Angles to Direction Cosine Matrix/1 -> Rotation Matrix to VRML Rotation1/1
  Rotation Matrix to VRML Rotation1/1 -> Out1/1

== system simulation/VR Mapping/Wheel positions to VRML/Build Rot Matrix3 ==
  In1 : Inport
  Constant1 : Constant  Value=pi/2
  Constant2 : Constant  Value=pi/2
  Mux : Mux  Inputs=3
  Rotation Angles to Direction Cosine Matrix : sharedtransform/Rotation Angles to Direction Cosine Matrix  rotationOrder=YZX  aMode=aMode
      settings: SourceProductBaseCode=AE
  Rotation Matrix to VRML Rotation1 : vrlib/Utilities/Rotation Matrix to VR Rotation  maxzero=1e-12
      settings: SourceProductName=Simulink 3D Animation  SourceProductBaseCode=VR
  Out1 : Outport  VectorParamsAs1DForOutWhenUnconnected=off
  wires:
  In1/1 -> Mux/1
  Mux/1 -> Rotation Angles to Direction Cosine Matrix/1
  Constant1/1 -> Mux/2
  Constant2/1 -> Mux/3
  Rotation Angles to Direction Cosine Matrix/1 -> Rotation Matrix to VRML Rotation1/1
  Rotation Matrix to VRML Rotation1/1 -> Out1/1

== system simulation/Model/Variant Subsystem/MPC/Extract reference vector ==
  In1 : Inport
  Increment Stored Integer : simulink/Additional Math & Discrete/Additional Math: Increment - Decrement/Increment Stored Integer
      settings: SourceProductName=Simulink
  Reshape : Reshape  OutputDimensions=1
  Selector : Selector  NumberOfDimensions=2  InputPortWidth=3  IndexOptions=Select all,Starting index (port)  Indices=[1 3],1  OutputSizes=1,MPC.nr
  Unit Delay : UnitDelay  InitialCondition=1  SampleTime=MPC.Ts  HasFrameUpgradeWarning=on
  Out1 : Outport  VectorParamsAs1DForOutWhenUnconnected=off
  wires:
  In1/1 -> Selector/1
  Unit Delay/1 -> Selector/2, Increment Stored Integer/1
  Increment Stored Integer/1 -> Unit Delay/1
  Selector/1 -> Reshape/1
  Reshape/1 -> Out1/1

== matlab function simulation/Model/Signal Packaging/MATLAB Function ==
  data: x input; dx output; dy output
function [dx,dy] = body_to_inertial_velocities(x)

phi = x(3);
R_EB = [cos(phi) -sin(phi);
            sin(phi) cos(phi)];

dxdy = R_EB*[x(5);x(6)];

dx = dxdy(1);
dy = dxdy(2);

== matlab function simulation/Model/Variant Subsystem/Feedback Linearised Position Control/MATLAB Function1 ==
  data: dw1 output; dw2 output; x input; w input; dtheta_pr output; theta_pr input; dxr input; dyr input; dphir input; fss_minus1_dvy_mvxdphi output
function [dw1,dw2,dtheta_pr,fss_minus1_dvy_mvxdphi] = get_dtheta_pr_dw1_dw2(x, w, theta_pr, dxr, dyr, dphir)

dw1 = 0;
dw2 = 0;
dtheta_pr = 0;
dvy_ss = 0;
fss_minus1_dvy_mvxdphi = 0;
theta_p_ss_error = 0;
% w1_0 = x(6)*x(7);


K_slow_dtheta_p = 0;
K_slow_theta_p = 20;
Kv = 6;
Kdphi = 0.1;

Kr = -150;
Kw1 = 50;
Kw2 = 150;

theta_p_max = 0.4;
w1_max = 3;
w2_max = 15;


% Calculate vxr vyr
phi = x(3);
R_EB = [cos(phi) -sin(phi);
            sin(phi) cos(phi)];
        
vxrvyr = R_EB'*[dxr;dyr];
vxr = vxrvyr(1);
vyr = vxrvyr(2);


% Calculate target steady state theta_p value for dvy=0 - remember this doesnt depend on v_y
fun = @(toSolve) f_solve_fdvy_theta_p_x([x(1:3);toSolve;x(5:7);0],zeros(3,1),-x(5)*x(7));
% fun = @(toSolve) f_solve_fdvy_theta_p_x([x(1:3);toSolve;x(5:7);0],[w(1);w(2);0],-vxr*dphir);


fss_minus1_dvy_mvxdphi = newtonRaphson(fun,0);

if fss_minus1_dvy_mvxdphi == theta_pr
    theta_pr = theta_pr + eps;
end

% % Calculate dvy_ss
% dvy_ss = dvy_ss_fun([x(1:3); theta_pr; x(5:8)]);


% Calculate rate of change of theta_p_ss due to dvx/w1 and ddphi/w2
% dfss_minus1_dvy_mvxdphi = solve_ddvy_ss_for_dthetapss_fun([x(1:3);fss_minus1_dvy_mvxdphi;x(5:7); 0], fss_minus1_dvy_mvxdphi, [w(1);w(2);0], (-w(1)*x(7) - w(2)*x(5)));
% dfss_minus1_dvy_mvxdphi = solve_ddvy_ss_for_dthetapss_fun([x(1:3);fss_minus1_dvy_mvxdphi;x(5:7); 0], fss_minus1_dvy_mvxdphi, [w(1);w(2);0], -vyr*dphir^2);

% Perform control
[dtheta_pr, dw1, dw2] = inertial_vel_control_dw1_dw2_dtheta_pr_fun(x, w, Kv, Kdphi, Kr, Kw1, Kw2, theta_p_max, w1_max, w2_max, theta_pr, dxr, dyr, dphir, fss_minus1_dvy_mvxdphi, K_slow_dtheta_p,K_slow_theta_p);


theta_p_ss_error = fss_minus1_dvy_mvxdphi - theta_pr;

% Slow outputs - now built-in
% dtheta_pr = dtheta_pr*exp(-10*abs(x(8)));
% dtheta_pr = dtheta_pr*exp(-20*abs(x(4)-theta_pr));


end

== matlab function simulation/Model/Variant Subsystem/Feedback Linearised Position Control/MATLAB Function ==
  data: x input; ddxr output; ref input; dref input; ddyr output; ddphir output
function [ddxr,ddyr,ddphir] = get_ddxr_ddyr_ddphir(x,ref,dref)

K_vr = 80;
K_p = 100;
K_dphir = 200;
K_phi = 1;
v_max = 1;
dphi_max = 6;

dxr = dref(1);
dyr = dref(2);
dphir = dref(3);
xr = ref(1);
yr = ref(2);
phir = ref(3);

K_slow = 20;

phi = x(3);
R_EB = [cos(phi) -sin(phi);
            sin(phi) cos(phi)];

dxdy = R_EB*[x(5); x(6);];
dx = dxdy(1);
dy = dxdy(2);


[ddxr,ddyr,ddphir] = inertial_pos_control_ddxr_ddyr_ddphir_fun(x,K_vr,K_p,K_dphir,K_phi,v_max,dphi_max,dxr,dyr,dphir,xr,yr,phir,K_slow);

== matlab function simulation/Model/Variant Subsystem/Feedback Linearised Body Velocity Control/MATLAB Function1 ==
  data: dw1 output; dw2 output; x input; w input; dtheta_pr output; theta_pr input; vxr input; vyr input; dphir input; fss_minus1_dvy0 output
function [dw1, dw2,dtheta_pr, fss_minus1_dvy0] = get_dtheta_pr_dw1_dw2(x, w, theta_pr, vxr, vyr, dphir)

coder.extrinsic('warning');

dw1 = 0;
dw2 = 0;
dtheta_pr = 0;
dvy_ss = 0;
w1 = 0;
fss_minus1_dvy0 = 0;

Kv = 4;
Kdphi = 0.1;

Kr = -60;
Kw1 = 5;
Kw2 = 150;
K_slow_dtheta_p = 0;
K_slow_theta_p = 20;

theta_p_max = 0.4;
w1_max = 3;
w2_max = 15;

% Calculate target steady state theta_p value for dvy=0 - remember this doesnt depend on v_y
fun = @(toSolve) f_solve_fdvy_theta_p_x([x(1:3);toSolve;x(5:7);0],zeros(3,1),0);
fss_minus1_dvy0 = newtonRaphson(fun,0);

if fss_minus1_dvy0 == theta_pr
    theta_pr = theta_pr + eps;
end

% Perform control
[dtheta_pr, dw1, dw2] = body_vel_control_dw1_dw2_dtheta_pr_fun(x, w, Kv, Kdphi, Kr, Kw1, Kw2, theta_p_max, w1_max, w2_max, theta_pr, fss_minus1_dvy0, vxr, vyr, dphir, K_slow_dtheta_p, K_slow_theta_p);


% dvy_ss = dvy_ss_fun([x(1:3); theta_pr; x(5:8)]);


end

== matlab function simulation/Model/Variant Subsystem/MPC/calculate_b ==
  data: x input; b output; r input; Fx input; Fr input; t input
function b = fcn(x, r, Fx, Fr, t)
    
b = t - Fx*x - Fr*r;

end

== matlab function simulation/Model/Variant Subsystem/Feedback Linearised Position Control/norm(v) ==
  data: x input; v output
function v = normv(x)

v = sqrt(x(1)^2 + x(2)^2);

== matlab function simulation/Model/Variant Subsystem/MPC/calculate_u ==
  data: u output; K input; Mx input; Drk1 input; Mu input; Dck input; Scr input; Sc input; x input; r input; c input
function u = fcn(K, Mx, Drk1, Mu, Dck, Scr, Sc, x, r, c)
    
 u = -K*x + (K*Mx + Mu)*Drk1*r + Dck*-(Sc\Scr)*r + Dck*c;

end

== matlab function simulation/Model/Variant Subsystem/Feedback Linearised Body Velocity Control/w due to rotation ==
  data: x input; dxdy output
function dxdy = fcn(x)

dxdy = [x(6)*x(7); -x(5)*x(7)];

== matlab function simulation/Model/Variant Subsystem/Feedback Linearised Inertial Velocity Control/FBL Inertial Velocity Controller ==
  data: dw1 output; dw2 output; x input; w input; dtheta_pr output; theta_pr input; dxr input; dyr input; dphir input; fss_minus1_dvy output; dxp output; dyp output
function [dw1,dw2,dtheta_pr,fss_minus1_dvy,dxp,dyp] = get_dtheta_pr_dw1_dw2(x, w, theta_pr, dxr, dyr, dphir)

dw1 = 0;
dw2 = 0;
dtheta_pr = 0;
dvy_ss = 0;
fss_minus1_dvy = 0;
theta_p_ss_error = 0;
dxp = 0;
dyp = 0;
    
% Two methods - original method, and differential flatness derived
% perturbation method
method = 1;
if method == 2

    K_slow_dtheta_p = 0;
    K_slow_theta_p = 10;
    Kvx = 0;
    Kvy = 0;
    Kdphi = 1;

    Kr = 0.1;
    Kw1 = 1;
    Kw2 = 150;

    theta_p_max = 0.6;
    w1_max = 3;
    w2_max = 15;

    % Calculate desired dvyp
    [dxp, dyp, ~, ~, dvxp, dvyp, ~, ~] = calculateInertialVelocityPerturbations(dxr, dyr, x(3), dphir);

    % and target theta_pss
    fun = @(toSolve) f_solve_fdvy_theta_p_x([x(1:3);toSolve;x(5:7);0],zeros(3,1),dvyp);
    fss_minus1_dvy_dvp = newtonRaphson(fun,0);

    if fss_minus1_dvy_dvp == theta_pr
        theta_pr = theta_pr + eps;
    end

    % % Calculate dvy_ss
    % dvy_ss = dvy_ss_fun([x(1:3); theta_pr; x(5:8)]);

    % Perform control
    [dtheta_pr, dw1, dw2] = inertial_vel_control_2_dw1_dw2_dtheta_pr_fun(x, w, Kvx, Kvy, Kdphi, Kr, Kw1, Kw2, theta_p_max, w1_max, w2_max, theta_pr, dxr, dyr, dphir, fss_minus1_dvy_dvp, K_slow_dtheta_p, K_slow_theta_p);

    theta_p_ss_error = fss_minus1_dvy_dvp - theta_pr;
    fss_minus1_dvy = fss_minus1_dvy_dvp;

elseif method == 1
    K_slow_dtheta_p = 0;
    K_slow_theta_p = 20;
    Kv = 4;
    Kdphi = 0.1;

    Kr = -150;
    Kw1 = 50;
    Kw2 = 150;

    theta_p_max = 0.4;
    w1_max = 3;
    w2_max = 15;


    % Calculate vxr vyr
    phi = x(3);
    R_EB = [cos(phi) -sin(phi);
                sin(phi) cos(phi)];

    vxrvyr = R_EB'*[dxr;dyr];
    vxr = vxrvyr(1);
    vyr = vxrvyr(2);


    % Calculate target steady state theta_p value for dvy=0 - remember this doesnt depend on v_y
    fun = @(toSolve) f_solve_fdvy_theta_p_x([x(1:3);toSolve;x(5:7);0],zeros(3,1),-x(5)*x(7));
    % fun = @(toSolve) f_solve_fdvy_theta_p_x([x(1:3);toSolve;x(5:7);0],[w(1);w(2);0],-vxr*dphir);


    fss_minus1_dvy_mvxdphi = newtonRaphson(fun,0);

    if fss_minus1_dvy_mvxdphi == theta_pr
        theta_pr = theta_pr + eps;
    end

    % % Calculate dvy_ss
    % dvy_ss = dvy_ss_fun([x(1:3); theta_pr; x(5:8)]);


    % Calculate rate of change of theta_p_ss due to dvx/w1 and ddphi/w2
    % dfss_minus1_dvy_mvxdphi = solve_ddvy_ss_for_dthetapss_fun([x(1:3);fss_minus1_dvy_mvxdphi;x(5:7); 0], fss_minus1_dvy_mvxdphi, [w(1);w(2);0], (-w(1)*x(7) - w(2)*x(5)));
    % dfss_minus1_dvy_mvxdphi = solve_ddvy_ss_for_dthetapss_fun([x(1:3);fss_minus1_dvy_mvxdphi;x(5:7); 0], fss_minus1_dvy_mvxdphi, [w(1);w(2);0], -vyr*dphir^2);

    % Perform control
    [dtheta_pr, dw1, dw2] = inertial_vel_control_dw1_dw2_dtheta_pr_fun(x, w, Kv, Kdphi, Kr, Kw1, Kw2, theta_p_max, w1_max, w2_max, theta_pr, dxr, dyr, dphir, fss_minus1_dvy_mvxdphi, K_slow_dtheta_p,K_slow_theta_p);


    theta_p_ss_error = fss_minus1_dvy_mvxdphi - theta_pr;
    fss_minus1_dvy = fss_minus1_dvy_mvxdphi;

    % Slow outputs - now built-in
    % dtheta_pr = dtheta_pr*exp(-10*abs(x(8)));
    % dtheta_pr = dtheta_pr*exp(-20*abs(x(4)-theta_pr));
end

end

== matlab function simulation/Model/Variant Subsystem/TVLQR/MATLAB Function ==
  data: x input; e output; xr input; e_i input
function e = e_fun(x,xr,e_i)


e = TVLQR_e_fun(x,xr,e_i);

== matlab function simulation/Model/Variant Subsystem/TVLQR/MATLAB Function1 ==
  data: tau_r input; x_r input; K output
function K = TVLQR(tau_r,x_r)

coder.extrinsic('lqr');

Q = blkdiag(eye(2), 0.01, eye(2), 0.01, zeros(5));
R = 1000*eye(numel(tau_r));

% Calculate A and B
A = TVLQR_A_fun(x_r,tau_r);
B = TVLQR_B_fun(x_r,tau_r);
K = zeros(size(B))';
K = lqr(A,B,Q,R);
K(:,1:3)=0;
% K(:,6)=0;


% % Remove integral
% A = A(4:end,4:end);
% B = B(4:end,:);
% Q = blkdiag(eye(3), zeros(5));
% 
% % Calculate LQR gain
% Knew = lqr(A,B,Q,R);
% K = [1*Knew(1:4,1:2) Knew(1:4,3) Knew];
